simulink model "simulare_lab_2"  (R2021b)
settings: Solver=VariableStepAuto  StartTime=0.0  StopTime=20.0  RelTol=1e-3
undefined symbols (not defined in the file or in its folder): x1, x2
settings Model: Creator=laurentiu  LastModifiedBy=laurentiu

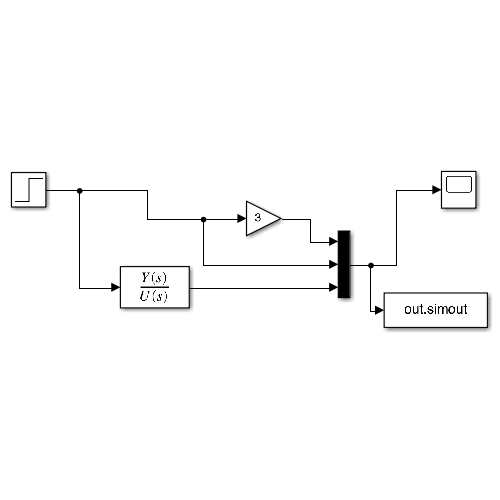
[thumbnail: Simulink's stored preview of the top-level diagram]
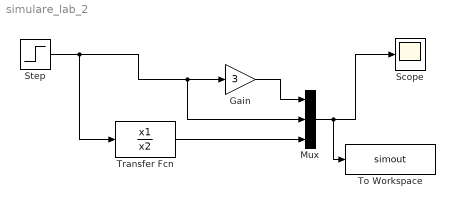
== system simulare_lab_2 ==
  Gain : Gain  Gain=3
  Mux : Mux  Inputs=3
  Scope : Scope
  Step : Step  Time=5  Before=2  After=4  SampleTime=0
  To Workspace : ToWorkspace  VariableName=simout  SaveFormat=Timeseries  SampleTime=-1
  Transfer Fcn : TransferFcn  Numerator=x1  Denominator=x2
  wires:
  Step/1 -> Transfer Fcn/1, Mux/2, Gain/1
  Gain/1 -> Mux/1
  Transfer Fcn/1 -> Mux/3
  Mux/1 -> To Workspace/1, Scope/1
